simulink model "Revised_model"  (Simulink 10.3)
settings: Solver=ode3  StartTime=0.0  StopTime=12  FixedStep=ts  MaxStep=1e-4  RelTol=1e-3
undefined symbols (not defined in the file or in its folder): Ion, Lithium, sigbuilder_block, ts
libraries: spsMeanLib x9, spsSeriesRLCBranchLib x6, spsIGBTDiodeLib x4, pid_lib x4, spsPWMGeneratorDCDCLib x4, spsBatteryLib x2, spsCurrentMeasurementLib x2, spsControlledCurrentSourceLib x2, spsVoltageMeasurementLib x2, spsFirstOrderFilterLib x1, spsDiodeLib x1, spsIGBTLib x1
(part 1 of 2)
settings Model: Creator=Rodayna  LastModifiedBy=Aditya  SimulationMode=accelerator
settings DataIOCC: SaveFormat=Dataset  SignalLoggingSaveFormat=Dataset
settings OptimizationCC: ExpressionDepthLimit=128  LifeSpan=auto
settings DebuggingCC: UnderspecifiedInitializationDetection=Simplified  MergeDetectMultiDrivingBlocksExec=error  FcnCallInpInsideContextMsg=error  StateNameClashWarn=none  SFUnexpectedBacktrackingDiag=error  SFNoUnconditionalDefaultTransitionDiag=error  SFExecutionAtInitializationDiag=warning
settings HardwareCC: ProdBitPerPointer=64  ProdBitPerSizeT=64  ProdBitPerPtrDiffT=64  ProdLargestAtomicFloat=Float  ProdIntDivRoundTo=Zero  ProdEndianess=LittleEndian  ProdWordSize=64  ProdHWDeviceType=Intel->x86-64 (Windows64)
settings ModelReferenceCC: PropagateSignalLabelsOutOfModel=on
settings GRTTargetCC: TargetLangStandard=C99 (ISO)  CombineOutputUpdateFcns=on  GRTInterface=off
settings ConfigComp: CovMetricSettings=dwe  CovSaveCumulativeToWorkspaceVar=off  CovSaveSingleToWorkspaceVar=off  CovExternalEMLEnable=on
settings SimscapeCC: SimscapeNormalizeSystem=off

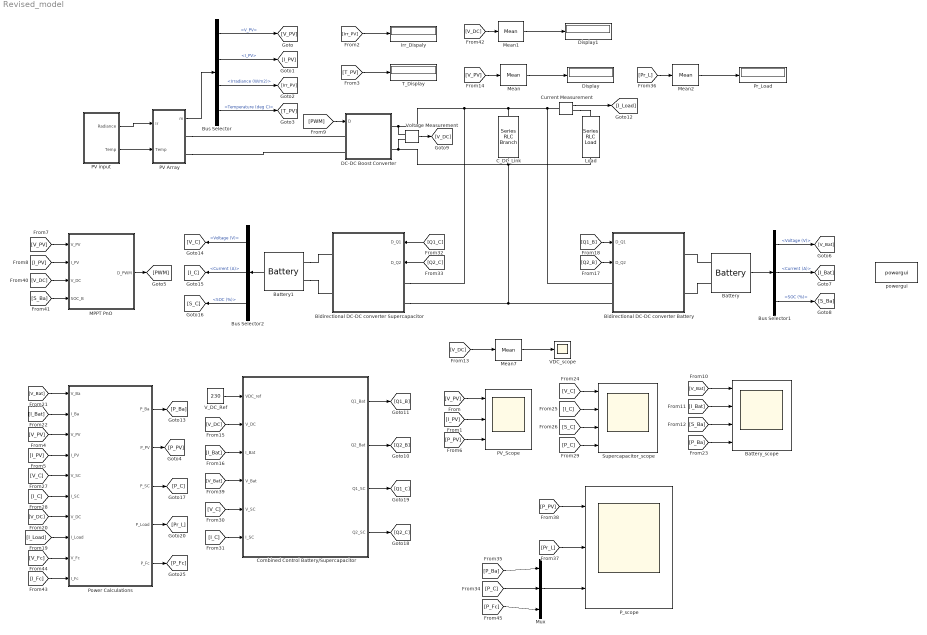
== system Revised_model ==
  Battery : spsBatteryLib/Battery  BatType=Lithium-Ion  ShowTempParam=off  ThermalPreset=no  ShowAgeParam=off  NomV=110  NomQ=150  SOC=50  Batt_Tr=0.1  PresetModel=on  MaxQ=150  MinV=82.5  FullV=128.0386  Dis_rate=65.2174  R=0.0073333  Normal_OP=135.6522  expZone="[118.8424      7.369565]"  current=[6.5 13 32.5]  Units=Time  Tci=20  NomT=20  T2=-30  MaxQ2=4.8  FullV2=7.1  Normal_OP2=5.655  expZone2="[6.58           1]"  Rca=0.6  ti=2000  Dp=0  Neq0=0  Tsim=1e6  Ta1=25  Qeol=5.4*0.9  Reol=0.013333*1.2  Char_age=[2.3478, 3]  Dis_age=[2.3478, 10]  N1=1500  N2=10500  N3=1000  N4=1400  Ta2=45  N5=950
  Battery1 : spsBatteryLib/Battery  BatType=Lithium-Ion  ShowTempParam=off  ThermalPreset=no  ShowAgeParam=off  NomV=154  NomQ=150  SOC=99  Batt_Tr=0.1  PresetModel=on  MaxQ=150  MinV=115.5  FullV=179.254  Dis_rate=65.2174  R=0.010267  Normal_OP=135.6522  expZone="[166.3794      7.369565]"  current=[6.5 13 32.5]  Units=Time  Tci=20  NomT=20  T2=-30  MaxQ2=4.8  FullV2=7.1  Normal_OP2=5.655  expZone2="[6.58           1]"  Rca=0.6  ti=2000  Dp=0  Neq0=0  Tsim=1e6  Ta1=25  Qeol=5.4*0.9  Reol=0.013333*1.2  Char_age=[2.3478, 3]  Dis_age=[2.3478, 10]  N1=1500  N2=10500  N3=1000  N4=1400  Ta2=45  N5=950
  "Battery_scope " : Scope  NumInputPorts=4
  Bidirectional DC-DC converter Battery : Subsystem
  Bidirectional DC-DC converter Supercapacitor : Subsystem
  Bus Selector : BusSelector  OutputSignals=V_PV,I_PV,Irradiance (W/m2),Temperature (deg C)
  Bus Selector1 : BusSelector  OutputSignals=Voltage (V),Current (A),SOC (%)
  Bus Selector2 : BusSelector  OutputSignals=Voltage (V),Current (A),SOC (%)
  C_DC_Link : spsSeriesRLCBranchLib/Series RLC Branch  LConnTagsString=__new0  RConnTagsString=__new0  BranchType=C  Resistance=1  Inductance=1e-3  SetiL0=off  InitialCurrent=0  Capacitance=3000e-6  Setx0=on  InitialVoltage=230  Measurements=None
  Combined Control Battery/Supercapacitor : Subsystem
  Current Measurement : spsCurrentMeasurementLib/Current Measurement  PhasorSimulation=off  OutputType=Complex  PSBequivalent=0
  DC-DC Boost Converter : Subsystem
  Display : Display
  Display1 : Display
  Irr_Dispaly : Display
  Load : spsSeriesRLCLoadLib/Series RLC Load  LConnTagsString=a  RConnTagsString=__new0  NominalVoltage=230  NominalFrequency=0.00001  ActivePower=10e3  InductivePower=0  CapacitivePower=0  Setx0=off  InitialVoltage=0  SetiL0=off  InitialCurrent=0  Measurements=None  LoadType=constant Z
  MPPT PnO : Subsystem
  Mean{,1..2,7} (4 alike) : spsMeanLib/Mean  Freq=60  Vinit=0  Ts=0
  Mux : Mux  Inputs=3
  PV Array : Subsystem  mask(PV array){ModuleType=BP Solar SX3190, Ncell=50, Nser=5, Npar=12, Voc=30.6021, Isc=8.5103, Vm=24.3003, Im=7.8294, TempC_Voc=-0.111, TempC_Isc=0.005532, TempC_Vmp=-0.114, TempC_Imp=-0.001566, Qd=1.25, Temperature=[0   25   50   75  100], Iph_Temp=[8.3797      8.5214       8.667      8.8096      8.9362], Isat_Temp=[1.1494e-09  4.3763e-08   9.524e-07  1.3432e-05  0.00013518], Rp_Temp=[479.1668      189.6748      120.6956      107.8176      267.7255], Rs_Temp=[0.24905     0.24841     0.25704     0.27792     0.31611], PlotVI_module=off, PlotVI_array=off, PlotVI_array_Temp=off, Ts=ts}
      mask prompts: ModuleType "Module type:"; Ncell "Number of cells per module:"; Nser "Number of series-connected  modules per string (Nser):"; Npar "Number of parallel strings (Npar):"; Voc "Open circuit voltage  Voc (V):"; Isc "Short-circuit current Isc (A):"; Vm "Voltage at maximum power point Vmp (V):"; Im "Current at maximum power point Imp (A):"; TempC_Voc "Temperature coefficient of Voc (V/deg.C)"; TempC_Isc "Temperature coefficient of Isc (A/deg.C)"; TempC_Vmp "Temperature coefficient of Vmp (V/deg.C)"; TempC_Imp "Temperature coefficient of Imp (A/deg.C"; Qd "Diode Quality factor"; Temperature "Cell temperature (degrees C)"; Iph_Temp "Photo-current source Iph  (A):"; Isat_Temp "Diode saturation current Isat (A):"; Rp_Temp "Parallel resistance Rp (ohms):"; Rs_Temp "Series resistance Rs (ohms):"; PlotVI_module "Display  I-V and  P-V characteristics of one module at 25 deg.C"; PlotVI_array "Display  I-V and  P-V characteristics of array at 25 deg.C"; PlotVI_array_Temp "Display  I-V and  P-V char. of array at 100W/m^2  for specified temperatures"; Ts "Sample time"
      mask help:
      | Model a PV array.
      |
      | PV array consists of Npar strings of modules connected in parallel, each string consisting of Nser modules connected in series.
      |
      | Input 1 = Sun irradiance (W/m^2)
      | Input 2 = Cell temperature (deg.C))
      |
      | Module specifications provided by manufacturer (Voc, Isc, Vmp, Imp) as well as temperature coefficients are listed under 'Module' Tab.
      | The four PV model parameters for one module (photo-generated current Iph, diode saturation current Isat, parallel resistance Rp and  series resistance Rs) are listed under the 'Model' Tab. These parameters are adusted to fit Voc, Isc, Vmp, Imp at specied cell temperatures listed under 'Module' Tab and assuming a given "diode quality factor" (Qd) for the semiconductor.
      |
      | Select a 'Module type' and then press Apply to see module parameters.
      | Note: Module characteristics are extracted from NREL System Advisor Model.
      mask init:
      | BlockName=gcb;
      | 
      | % Solar Modules Specifications
      | %=============================
      | %
      | Type=1;
      | SolarModuleSpec(Type).Desc= 'Kyocera KD135GX-LP';
      | SolarModuleSpec(Type).nCells= 36;
      | SolarModuleSpec(Type).Voc= 22.0999;
      | SolarModuleSpec(Type).Isc= 8.36955;
      | SolarModuleSpec(Type).Vmp= 17.7;
      | SolarModuleSpec(Type).Imp= 7.62959;
      | SolarModuleSpec(Type).TempC_Voc= -0.08;
      | SolarModuleSpec(Type).TempC_Isc= 0.005022;
      | SolarModuleSpec(Type).TempC_Vmp= -0.082;
      | SolarModuleSpec(Type).TempC_Imp= -0.001068;
      | SolarModuleSpec(Type).TempC= [0   25   50   75  100];
      | SolarModuleSpec(Type).Qd= 1.25;
      | SolarModuleSpec(Type).Iph= [8.2548      8.3863      8.5179      8.6475      8.7657];
      | SolarModuleSpec(Type).Isat= [1.0452e-09  4.0088e-08  8.7854e-07   1.246e-05  0.00012585];
      | SolarModuleSpec(Type).Rp= [124.2147      80.21788      61.82143      57.59975       93.2949];
      | SolarModuleSpec(Type).Rs= [0.16273     0.16086     0.16567     0.17914     0.20462];
      | SolarModuleSpec(Type).VT= [1.0586      1.1555      1.2525      1.3494      1.4463];
      | 
      | Type=2;
      | SolarModuleSpec(Type).Desc= 'Kyocera KD205GX-LP';
      | SolarModuleSpec(Type).nCells= 54;
      | SolarModuleSpec(Type).Voc= 33.1999;
      | SolarModuleSpec(Type).Isc= 8.35955;
      | SolarModuleSpec(Type).Vmp= 26.6;
      | SolarModuleSpec(Type).Imp= 7.70959;
      | SolarModuleSpec(Type).TempC_Voc= -0.12;
      | SolarModuleSpec(Type).TempC_Isc= 0.005016;
      | SolarModuleSpec(Type).TempC_Vmp= -0.123;
      | SolarModuleSpec(Type).TempC_Imp= -0.001079;
      | SolarModuleSpec(Type).TempC= [0   25   50   75  100];
      | SolarModuleSpec(Type).Qd= 1.5;
      | SolarModuleSpec(Type).Iph= [8.2611      8.3642      8.4897      8.6397      8.8494];
      | SolarModuleSpec(Type).Isat= [4.6184e-08  9.7399e-07  1.2856e-05  0.00011784  0.00080899];
      | SolarModuleSpec(Type).Rp= [1053.4598       1010.571      746.03259      733.82072      575.51725];
      | SolarModuleSpec(Type).Rs= [0.16179     0.15945     0.16818     0.19126     0.23373];
      | SolarModuleSpec(Type).VT= [1.9055      2.0799      2.2544      2.4289      2.6034];
      | 
      | Type=3;
      | SolarModuleSpec(Type).Desc= 'Mitsubishi PV-UD190MF5';
      | SolarModuleSpec(Type).nCells= 50;
      | SolarModuleSpec(Type).Voc= 30.8006;
      | SolarModuleSpec(Type).Isc= 8.23289;
      | SolarModuleSpec(Type).Vmp= 24.6999;
      | SolarModuleSpec(Type).Imp= 7.71272;
      | SolarModuleSpec(Type).TempC_Voc= -0.105;
      | SolarModuleSpec(Type).TempC_Isc= 0.004446;
      | SolarModuleSpec(Type).TempC_Vmp= -0.109;
      | SolarModuleSpec(Type).TempC_Imp= -0.0007713;
      | SolarModuleSpec(Type).TempC= [0   25   50   75  100];
      | SolarModuleSpec(Type).Qd= 1.25;
      | SolarModuleSpec(Type).Iph= [8.1758      8.2585      8.3644      8.4965      8.6704];
      | SolarModuleSpec(Type).Isat= [1.0882e-09  3.8061e-08  7.7001e-07  1.0166e-05  9.5622e-05];
      | SolarModuleSpec(Type).Rp= [760.17338      1011.1501      920.18116      953.25748       1044.703];
      | SolarModuleSpec(Type).Rs= [0.22154      0.2231     0.23302     0.25351     0.28829];
      | SolarModuleSpec(Type).VT= [1.4703      1.6049      1.7395      1.8742      2.0088];
      | 
      | Type=4;
      | SolarModuleSpec(Type).Desc= 'Sanyo HIP-225HDE1';
      | SolarModuleSpec(Type).nCells= 60;
      | SolarModuleSpec(Type).Voc= 41.7984;
      | SolarModuleSpec(Type).Isc= 7.13383;
      | SolarModuleSpec(Type).Vmp= 33.9;
      | SolarModuleSpec(Type).Imp= 6.63419;
      | SolarModuleSpec(Type).TempC_Voc= -0.105;
      | SolarModuleSpec(Type).TempC_Isc= 0.00214;
      | SolarModuleSpec(Type).TempC_Vmp= -0.101;
      | SolarModuleSpec(Type).TempC_Imp= -0.0006634;
      | SolarModuleSpec(Type).TempC= [0   25   50   75  100];
      | SolarModuleSpec(Type).Qd= 1.75;
      | SolarModuleSpec(Type).Iph= [7.1125      7.1668      7.2277      7.3002      7.3835];
      | SolarModuleSpec(Type).Isat= [1.0956e-07   1.322e-06  1.0873e-05  6.6227e-05  0.00031754];
      | SolarModuleSpec(Type).Rp= [1677.488      1798.4952      1967.0424      1956.9124      2053.1618];
      | SolarModuleSpec(Type).Rs= [0.19173     0.14196     0.10096    0.069476    0.049098];
      | SolarModuleSpec(Type).VT= [2.47      2.6962      2.9224      3.1486      3.3748];
      | 
      | Type=5;
      | SolarModuleSpec(Type).Desc= 'SunPower SPR-305-WHT';
      | SolarModuleSpec(Type).nCells= 96;
      | SolarModuleSpec(Type).Voc= 64.2;
      | SolarModuleSpec(Type).Isc= 5.96;
      | SolarModuleSpec(Type).Vmp= 54.7;
      | SolarModuleSpec(Type).Imp= 5.58;
      | SolarModuleSpec(Type).TempC_Voc= -0.177;
      | SolarModuleSpec(Type).TempC_Isc= 0.003516;
      | SolarModuleSpec(Type).TempC_Vmp= -0.186;
      | SolarModuleSpec(Type).TempC_Imp= -0.00212;
      | SolarModuleSpec(Type).TempC= [0   25   50   75  100];
      | SolarModuleSpec(Type).Qd= 1.25;
      | SolarModuleSpec(Type).Iph= [5.9045      5.9606      6.0494      6.1386      6.2292];
      | SolarModuleSpec(Type).Isat= [1.6236e-10  5.2622e-09  9.8888e-08  1.2201e-06  1.0769e-05];
      | SolarModuleSpec(Type).Rp= [1723.2701      819.13001       313.3225      186.86379      130.70398];
      | SolarModuleSpec(Type).Rs= [0.10187    0.083029    0.075997    0.085738      0.1163];
      | SolarModuleSpec(Type).VT= [2.8229      3.0814      3.3399      3.5984      3.8569];
      | 
      | Type=6;
      | SolarModuleSpec(Type).Desc= 'Suntech STP270S-24_Vb';
      | SolarModuleSpec(Type).nCells= 72;
      | SolarModuleSpec(Type).Voc= 44.4999;
      | SolarModuleSpec(Type).Isc= 8.19978;
      | SolarModuleSpec(Type).Vmp= 35;
      | SolarModuleSpec(Type).Imp= 7.70979;
      | SolarModuleSpec(Type).TempC_Voc= -0.1504;
      | SolarModuleSpec(Type).TempC_Isc= 0.004969;
      | SolarModuleSpec(Type).TempC_Vmp= -0.1567;
      | SolarModuleSpec(Type).TempC_Imp= 0.0001234;
      | SolarModuleSpec(Type).TempC= [0   25   50   75  100];
      | SolarModuleSpec(Type).Qd= 1.25;
      | SolarModuleSpec(Type).Iph= [8.1345      8.2466      8.3792      8.5437      8.7583];
      | SolarModuleSpec(Type).Isat= [1.0212e-09   3.569e-08  7.2273e-07  9.5489e-06  8.9954e-05];
      | SolarModuleSpec(Type).Rp= [1505.3115      1827.4593      2300.9307      2164.0121      1763.1975];
      | SolarModuleSpec(Type).Rs= [0.4218     0.42722     0.44553     0.48023      0.5376];
      | SolarModuleSpec(Type).VT= [2.1172      2.3111      2.5049      2.6988      2.8927];
      | 
      | Type=7;
      | SolarModuleSpec(Type).Desc= 'Canadian Solar CS5P-220M';
      | SolarModuleSpec(Type).nCells= 96;
      | SolarModuleSpec(Type).Voc= 59.2618;
      | SolarModuleSpec(Type).Isc= 5.09261;
      | SolarModuleSpec(Type).Vmp= 48.3159;
      | SolarModuleSpec(Type).Imp= 4.54758;
      | SolarModuleSpec(Type).TempC_Voc= -0.217;
      | SolarModuleSpec(Type).TempC_Isc= 0.002022;
      | SolarModuleSpec(Type).TempC_Vmp= -0.2355;
      | SolarModuleSpec(Type).TempC_Imp= 0.0008231;
      | SolarModuleSpec(Type).TempC= [0   25   50   75  100];
      | SolarModuleSpec(Type).Qd= 1.5;
      | SolarModuleSpec(Type).Iph= [5.046       5.098      5.1493      5.1959      5.3427];
      | SolarModuleSpec(Type).Isat= [2.4207e-08  5.3103e-07  7.2907e-06  6.9747e-05  0.00049283];
      | SolarModuleSpec(Type).Rp= [222.52442      235.76261      303.25525      1307.0023      2378.4408];
      | SolarModuleSpec(Type).Rs= [0.17441     0.24807     0.36157     0.52616      0.7509];
      | SolarModuleSpec(Type).VT= [3.3875      3.6977      4.0079      4.3181      4.6283];
      | 
      | Type=8;
      | SolarModuleSpec(Type).Desc= 'BP Solar SX3190';
      | SolarModuleSpec(Type).nCells= 50;
      | SolarModuleSpec(Type).Voc= 30.6021;
      | SolarModuleSpec(Type).Isc= 8.51029;
      | SolarModuleSpec(Type).Vmp= 24.3003;
      | SolarModuleSpec(Type).Imp= 7.82945;
      | SolarModuleSpec(Type).TempC_Voc= -0.111;
      | SolarModuleSpec(Type).TempC_Isc= 0.005532;
      | SolarModuleSpec(Type).TempC_Vmp= -0.114;
      | SolarModuleSpec(Type).TempC_Imp= -0.001566;
      | SolarModuleSpec(Type).TempC= [0   25   50   75  100];
      | SolarModuleSpec(Type).Qd= 1.25;
      | SolarModuleSpec(Type).Iph= [8.3797      8.5214       8.667      8.8096      8.9362];
      | SolarModuleSpec(Type).Isat= [1.1494e-09  4.3763e-08   9.524e-07  1.3432e-05  0.00013518];
      | SolarModuleSpec(Type).Rp= [479.1668      189.6748      120.6956      107.8176      267.7255];
      | SolarModuleSpec(Type).Rs= [0.24905     0.24841     0.25704     0.27792     0.31611];
      | SolarModuleSpec(Type).VT= [1.4703      1.6049      1.7395      1.8742      2.0088];
      | 
      | Type=9;
      | SolarModuleSpec(Type).Desc= 'First Solar FS-272';
      | SolarModuleSpec(Type).nCells= 116;
      | SolarModuleSpec(Type).Voc= 94.5738;
      | SolarModuleSpec(Type).Isc= 1.18103;
      | SolarModuleSpec(Type).Vmp= 70.558;
      | SolarModuleSpec(Type).Imp= 1.01088;
      | SolarModuleSpec(Type).TempC_Voc= -0.269;
      | SolarModuleSpec(Type).TempC_Isc= 0.0005433;
      | SolarModuleSpec(Type).TempC_Vmp= -0.206;
      | SolarModuleSpec(Type).TempC_Imp= -0.0003538;
      | SolarModuleSpec(Type).TempC= [0   25   50   75  100];
      | SolarModuleSpec(Type).Qd= 3;
      | SolarModuleSpec(Type).Iph= [1.1706      1.1841      1.1969       1.209      1.2204];
      | SolarModuleSpec(Type).Isat= [4.7807e-06   2.871e-05  0.00013082  0.00048055    0.001489];
      | SolarModuleSpec(Type).Rp= [2555.993      1859.5401      1459.3976      1213.5712      1072.4965];
      | SolarModuleSpec(Type).Rs= [6.9861      4.7977      2.7078     0.74048           0];
      | SolarModuleSpec(Type).VT= [8.1864      8.93607      9.68574      10.4354      11.1851];
      | 
      | Type=10;
      | SolarModuleSpec(Type).Desc= 'SunPower 128-cell Module';
      | SolarModuleSpec(Type).nCells= 128;
      | SolarModuleSpec(Type).Voc= 85.2983;
      | SolarModuleSpec(Type).Isc= 5.8675;
      | SolarModuleSpec(Type).Vmp= 72.8992;
      | SolarModuleSpec(Type).Imp= 5.48769;
      | SolarModuleSpec(Type).TempC_Voc= -0.2664;
      | SolarModuleSpec(Type).TempC_Isc= 0.001837;
      | SolarModuleSpec(Type).TempC_Vmp= -0.276;
      | SolarModuleSpec(Type).TempC_Imp= -0.00169;
      | SolarModuleSpec(Type).TempC= [0   25   50   75  100];
      | SolarModuleSpec(Type).Qd= 1.5;
      | SolarModuleSpec(Type).Iph= [5.8403      5.8693      5.9126      5.9583      6.0069];
      | SolarModuleSpec(Type).Isat= [8.3639e-09  1.7905e-07  2.3847e-06  2.1965e-05  0.00015113];
      | SolarModuleSpec(Type).Rp= [3739.8323      3390.2471      1695.8516      1327.4043      1910.4252];
      | SolarModuleSpec(Type).Rs= [0  0  0  0  0];
      | SolarModuleSpec(Type).VT= [4.5166      4.9302      5.3439      5.7575      6.1711];
      | 
      | 
      | %-------------------------------------------------------------------------
      | 
      | Type=strmatch(ModuleType,char(SolarModuleSpec.Desc));
      | 
      | % Write module prameters inside mask
      | %===================================
      | set_param(BlockName,'Ncell',num2str(SolarModuleSpec(Type).nCells));
      | set_param(BlockName,'Voc',num2str(SolarModuleSpec(Type).Voc));
      | set_param(BlockName,'Isc',num2str(SolarModuleSpec(Type).Isc));
      | set_param(BlockName,'Vm',num2str(SolarModuleSpec(Type).Vmp));
      | set_param(BlockName,'Im',num2str(SolarModuleSpec(Type).Imp));
      | set_param(BlockName,'TempC_Voc',num2str(SolarModuleSpec(Type).TempC_Voc));
      | set_param(BlockName,'TempC_Isc',num2str(SolarModuleSpec(Type).TempC_Isc));
      | set_param(BlockName,'TempC_Vmp',num2str(SolarModuleSpec(Type).TempC_Vmp));
      | set_param(BlockName,'TempC_Imp',num2str(SolarModuleSpec(Type).TempC_Imp));
      | 
      | set_param(BlockName,'Qd',num2str(SolarModuleSpec(Type).Qd));
      | 
      | set_param(BlockName,'Temperature',['[',num2str(SolarModuleSpec(Type).TempC),']']);
      | set_param(BlockName,'Iph_Temp',['[',num2str(SolarModuleSpec(Type).Iph),']']);
      | set_param(BlockName,'Isat_Temp',['[',num2str(SolarModuleSpec(Type).Isat),']']);
      | set_param(BlockName,'Rp_Temp',['[',num2str(SolarModuleSpec(Type).Rp),']']);
      | set_param(BlockName,'Rs_Temp',['[',num2str(SolarModuleSpec(Type).Rs),']']);
      | 
      | TC=25; % standard test temperature (deg. C)
      | T=273+TC; %(Kelvin)
      | nT=find(SolarModuleSpec(Type).TempC==TC);
      | 
      | % Array model parameters
      | %=======================
      | % Qd=SolarModuleSpec(Type).Qd;
      | % k= 1.3806e-23; % Boltzman constant (J.K^-1)
      | % q=1.6022e-19;  % electron charge  (C)
      | % VT=k*T/q*nCells*Qd;
      | VT=SolarModuleSpec(Type).VT(nT);Iph=SolarModuleSpec(Type).Iph(nT); 
      | 
      | TempC=SolarModuleSpec(Type).TempC;
      | Iph_array=SolarModuleSpec(Type).Iph*Npar;
      | Isat_array=SolarModuleSpec(Type).Isat*Npar;
      | VT_array=SolarModuleSpec(Type).VT*Nser;
      | Rs_array=SolarModuleSpec(Type).Rs*Nser/Npar;
      | Rp_array=SolarModuleSpec(Type).Rp*Nser/Npar;
      | 
      | % Used to determine initial value of Boost Control (MPPT)
      | % assignin('base','Vm_Init',Vm*Nser);
      | %
      | % Plot module and array I-V & P-V characteristics for different irradiances
      | % =========================================================================
      | if PlotVI_module || PlotVI_array 
      |     Voc=SolarModuleSpec(Type).Voc; 
      |     Isc=SolarModuleSpec(Type).Isc; 
      |     Vm=SolarModuleSpec(Type).Vmp;  
      |     Im=SolarModuleSpec(Type).Imp;
      |     
      |     load_system('PV_model_Param');
      |     
      |     assignin('base','Voc',Voc);
      |     assignin('base','Isc',Isc);
      |     assignin('base','Rs',SolarModuleSpec(Type).Rs(nT));
      |     assignin('base','Rp',SolarModuleSpec(Type).Rp(nT));
      |     assignin('base','Isat',SolarModuleSpec(Type).Isat(nT));
      |     assignin('base','VT',SolarModuleSpec(Type).VT(nT));
      |    
      |     if PlotVI_module,
      |         F1=figure('Name','I-V and P-V characteristics of one module at 25 deg.C');  
      |     end
      |     if PlotVI_array
      |         F2=figure('Name','I-V and P-V characteristics of array at 25 deg.C'); 
      |     end
      | 
      |     for ksun=1:-0.25:0.25
      |         assignin('base','Iph',SolarModuleSpec(Type).Iph(nT)*ksun);
      |         sim('PV_model_Param');
      |         n=find(I_PV>=0);
      |         I_PV=I_PV(n);
      |         V_PV=V_PV(n);
      |         P_PV=V_PV.*I_PV;
      |         
      |         % Plot I-V & P-V characteristics of one module
      |         %=============================================
      |         if PlotVI_module
      |             figure(F1);
      |             subplot(211)
      |             if ksun==1
      |                 plot(V_PV,I_PV,'b',[0  Vm Voc], [Isc Im 0],'ro')
      |                 text(Voc/15,Isc*1.1,'1 kW/m^2')
      |                 hold on
      |                 grid
      |             else
      |                 plot(V_PV,I_PV,'--m')
      |                 text(Voc/15, Isc*(ksun+0.1) , sprintf('%g kW/m^2',ksun))
      |             end
      | 
      |             subplot(212) 
      |             if ksun==1
      |                 plot(V_PV,P_PV,'b',[0  Vm Voc], [0 Im*Vm 0],'ro')
      |                 text(Vm*1.02,Vm*Im,'1 kW/m^2')
      |                 hold on
      |                 grid
      |             else
      |                 n= find(P_PV==max(P_PV));
      |                 plot(V_PV,P_PV,'--m', V_PV(n) , P_PV(n),'mo')
      |                 text(Vm*1.02, Vm*Im*ksun, sprintf('%g kW/m^2',ksun))
      |             end
      |             subplot(211)
      |             ylabel('Current (A)')
      |             xlabel('Voltage (V)')
      |             title(sprintf('Module type: %s',SolarModuleSpec(Type).Desc))
      |             axis_xy=axis;
      |             axis_xy(4)=Isc*1.2;
      |             axis(axis_xy);
      |             
      |             subplot(212)
      |             ylabel('Power (W)')
      |             xlabel('Voltage (V)')
      |             axis_xy=axis;
      |             axis_xy(4)=Vm*Im*1.2;
      |             axis(axis_xy);
      |                   
      |             set_param(BlockName,'PlotVI_module', 'off')
      |         end
      |         
      |         % Plot I-V & P-V characteristics of array
      |         %========================================
      |         if PlotVI_array
      |             figure(F2);
      |             subplot(211)
      |             if ksun==1
      |                 plot(V_PV*Nser,I_PV*Npar,'b',[0  Vm Voc]*Nser, [Isc Im 0]*Npar,'ro')
      |                 text(Voc/15*Nser,Isc*1.1*Npar,'1 kW/m^2')
      |                 hold on
      |                 grid
      |             else
      |                 plot(V_PV*Nser,I_PV*Npar,'--m')
      |                 text(Voc*Nser/15, Isc*Npar*(ksun+0.1) , sprintf('%g kW/m^2',ksun))
      |             end
      |            
      |             subplot(212)
      |             if ksun==1
      |                 plot(V_PV*Nser,P_PV*Nser*Npar,'b',[0  Vm Voc]*Nser, [0 Im*Vm 0]*Nser*Npar,'ro')
      |                 text(Vm*Nser*1.02,Vm*Im*Nser*Npar,'1 kW/m^2')
      |                 hold on
      |                 grid
      |             else
      |                 n= find(P_PV==max(P_PV));
      |                 plot(V_PV*Nser,P_PV*Nser*Npar,'--m', V_PV(n)*Nser , P_PV(n)*Nser*Npar,'mo')
      |                 text(Vm*Nser*1.02, Vm*Im*Nser*Npar*ksun, sprintf('%g kW/m^2',ksun))
      |             end 
      |             subplot(211)
      |             ylabel('Current (A)')
      |             xlabel('Voltage (V)')
      |             title(sprintf('Array type: %s; %d series modules; %d parallel strings',SolarModuleSpec(Type).Desc,Nser,Npar));
      |             axis_xy=axis;
      |             axis_xy(4)=Isc*Npar*1.2;
      |             axis(axis_xy);
      |             
      |             subplot(212)
      |             ylabel('Power (W)')
      |             xlabel('Voltage (V)')
      |             xis_xy=axis;
      |             axis_xy(4)=Vm*Im*Nser*Npar*1.2;
      |             axis(axis_xy);
      |             
      |             set_param(BlockName,'PlotVI_array', 'off')
      |         end
      |         
      |     end  
      | end
      | 
      | %%  Plot array V-I & P_V characteristics for different temperatures
      | % =================================================================
      | if PlotVI_array_Temp
      |     F3=figure('Name',' I-V and P-V characteristics of array at 1000 W/m^2');
      |     load_system('PV_model_Param');
      |     for ktemp=1:length(TempC)
      |         DeltaT=TempC(ktemp)-25;
      |         Voc=SolarModuleSpec(Type).Voc + SolarModuleSpec(Type).TempC_Voc*DeltaT;
      |         Isc=SolarModuleSpec(Type).Isc + SolarModuleSpec(Type).TempC_Isc*DeltaT;
      |         Vm=SolarModuleSpec(Type).Vmp  + SolarModuleSpec(Type).TempC_Vmp*DeltaT;
      |         Im=SolarModuleSpec(Type).Imp  + SolarModuleSpec(Type).TempC_Imp*DeltaT;
      | 
      |         assignin('base','Voc',Voc)
      |         assignin('base','Isc',Isc)
      |         assignin('base','Iph',SolarModuleSpec(Type).Iph(ktemp));
      |         assignin('base','Isat',SolarModuleSpec(Type).Isat(ktemp));
      |         assignin('base','Rs',SolarModuleSpec(Type).Rs(ktemp));
      |         assignin('base','Rp',SolarModuleSpec(Type).Rp(ktemp));
      |         assignin('base','VT',SolarModuleSpec(Type).VT(ktemp));
      |         
      |         sim('PV_model_Param');
      |         n=find(I_PV>=0);
      |         I_PV=I_PV(n);
      |         V_PV=V_PV(n);
      |         P_PV=V_PV.*I_PV;
      | 
      |         subplot(211)
      |         if TempC(ktemp)==25
      |             plot(V_PV*Nser,I_PV*Npar,'b',[0  Vm Voc]*Nser, [Isc Im 0]*Npar,'ro')
      |             text(Voc*Nser*0.95, Isc*Npar/10*(1+ktemp) , sprintf('%g ^oC',TempC(ktemp)))
      |             %hold on
      |             grid
      |         else
      |             plot(V_PV*Nser,I_PV*Npar,'--m',[0  Vm Voc]*Nser, [Isc Im 0]*Npar,'mo')
      |             text(Voc*Nser*0.95, Isc*Npar/10*(1+ktemp) , sprintf('%g ^oC',TempC(ktemp)))
      |         end
      |         if ktemp==1, hold on; end
      | 
      |         subplot(212) 
      |         if TempC(ktemp)==25
      |             plot(V_PV*Nser,P_PV*Nser*Npar,'b',[0  Vm Voc]*Nser, [0 Im*Vm 0]*Nser*Npar,'ro')
      |             text(Vm*Nser, 0.9*Vm*Im*Nser*Npar , sprintf('%g ^oC',TempC(ktemp)))
      |             %hold on
      |             grid
      |         else
      |             n= find(P_PV==max(P_PV));
      |             plot(V_PV*Nser,P_PV*Nser*Npar,'--m', V_PV(n)*Nser , P_PV(n)*Nser*Npar,'mo')
      |             text(Vm*Nser, 0.9*Vm*Im*Nser*Npar , sprintf('%g ^oC',TempC(ktemp)))
      |         end
      |         if ktemp==1, hold on; end
      |     end
      |         
      |     subplot(211)
      |     ylabel('Current (A)')
      |     xlabel('Voltage (V)')
      |     title(sprintf('Array type: %s; %d series modules; %d parallel strings',SolarModuleSpec(Type).Desc,Nser,Npar));
      |     subplot(212)
      |     ylabel('Power (W)')
      |     xlabel('Voltage (V)')
      |     set_param(BlockName,'PlotVI_array_Temp', 'off')
      | end
      mask TypeOptions ModuleType: BP Solar SX3190 | Canadian Solar CS5P-220M | First Solar FS-272 | Kyocera KD135GX-LP | Kyocera KD205GX-LP | Mitsubishi PV-UD190MF5 | Sanyo HIP-225HDE1 | SunPower SPR-305-WHT | SunPower SPR-400-WHT | Suntech STP270S-24_Vb
      mask Display: image(imread('panel.jpg'))
  PV input : Subsystem  Tag=STV Subsys  LoadFcn=sigbuilder_block('load');  StartFcn=sigbuilder_block('start');  StopFcn=sigbuilder_block('stop');  ClipboardFcn=sigbuilder_block('clipboard');  mask(Sigbuilder block){tuvar=[0:10]}
      mask help: Simulink:masks:SigbuilderBlock_MD
      mask init:
      | if ~strcmp(get_param(bdroot(gcbh),'SimulationStatus'),'stopped') tuvar = sigbuilder_block('maskInit'); end
      settings: CopyFcn=sigbuilder_block('copy');  DeleteFcn=sigbuilder_block('delete');  ModelCloseFcn=sigbuilder_block('modelClose');  PreSaveFcn=sigbuilder_block('preSave');  PauseFcn=sigbuilder_block('pause');  ContinueFcn=sigbuilder_block('continue');  NameChangeFcn=sigbuilder_block('namechange');  OpenFcn=sigbuilder_block('open',[437.25 117.75 550.5 394.5 ]);  CloseFcn=sigbuilder_block('close');
      mask Display: plot(0, 0, 100, 100,[2, 2, 32, 32, 2], [68, 8, 8, 68, 68],[32, 2], [38, 38], [32, 19, 2],[53, 60, 44], [32, 17, 17, 2],[16, 16, 31, 31]);txt = getActiveGroup(gcbh);text(2, 100, txt,'verticalAlignment', 'top');
  PV_Scope : Scope  NumInputPorts=3
  P_scope : Scope  NumInputPorts=3
  Power Calculations : Subsystem
  Pr_Load : Display
  Supercapacitor_scope : Scope  NumInputPorts=4
  T_Display : Display
  VDC_scope : Scope
  V_DC_Ref : Constant  Value=230
  Voltage Measurement : spsVoltageMeasurementLib/Voltage Measurement  PhasorSimulation=off  OutputType=Complex  PSBequivalent=0
  powergui : spspowerguiLib/powergui  Priority=1  SimulationMode=Discrete  SampleTime=ts  frequency=60  Iterations=50  frequencyindice=0  Pbase=100e6  ErrMax=1e-4  UnitsV=kV  UnitsW=MW  buscounter=0  FunctionMessages=off  echomessages=off  EnableUseOfTLC=off  CurrentSourceSwitches=off  DisableSnubberDevices=off  DisableRonSwitches=off  DisableVfSwitches=off  DisplayEquations=off  AutomaticDiscreteSolvers=off  SolverType=Tustin/Backward Euler (TBE)  Interpol=off  ExternalGateDelay=off  methode=off  Ts=100  x0status=blocks  SPID=on  SwTol=0  HookPort=off  NonlinearTolerance=1e-4  nMaxIteration=100  ContinueOnMaxIteration=off  RestoreLinks=warning  ResistiveCurrentMeasurement=off  Frange=[0:2:500]  Ylog=off  Xlog=on  ShowGrid=off  save=off  variable=ZData  structure=0  ZoomFFT=off  StartTime=0.0  cycles=1  DisplayStyle=1  fundamental=60  FreqAxis=off  MaxFrequency=1000  frequencyindicesteady=1  RmsSteady=1  display=off
  wires:
  PV Array/1(m) -> Bus Selector/1
  Bus Selector/1 -> [V_PV]  "<V_PV>"
  Bus Selector/2 -> [I_PV]  "<I_PV>"
  Bus Selector/3 -> [Irr_PV]  "<Irradiance (W/m2)>"
  Bus Selector/4 -> [T_PV]  "<Temperature (deg C)>"
  [Irr_PV] -> Irr_Dispaly/1
  [T_PV] -> T_Display/1
  [PWM] -> DC-DC Boost Converter/1(D)
  [V_PV] -> MPPT PnO/1(V_PV)
  [I_PV] -> MPPT PnO/2(I_PV)
  MPPT PnO/1(D_PWM) -> [PWM]
  Battery/1 -> Bus Selector1/1
  Bus Selector1/1 -> [V_Bat]  "<Voltage (V)>"
  Bus Selector1/3 -> [S_Ba]  "<SOC (%)>"
  Bus Selector1/2 -> [I_Bat]  "<Current (A)>"
  Voltage Measurement/1 -> [V_DC]
  [Q2_B] -> Bidirectional DC-DC converter Battery/2(D_Q2)
  [Q1_B] -> Bidirectional DC-DC converter Battery/1(D_Q1)
  Current Measurement/1 -> [I_Load]
  Mean/1 -> Display/1
  [V_PV] -> Mean/1
  Mean1/1 -> Display1/1
  Battery1/1 -> Bus Selector2/1
  Bus Selector2/1 -> [V_C]  "<Voltage (V)>"
  Bus Selector2/2 -> [I_C]  "<Current (A)>"
  Bus Selector2/3 -> [S_C]  "<SOC (%)>"
  [Q1_C] -> Bidirectional DC-DC converter Supercapacitor/1(D_Q1)
  [Q2_C] -> Bidirectional DC-DC converter Supercapacitor/2(D_Q2)
  Mean2/1 -> Pr_Load/1
  [Pr_L] -> Mean2/1
  PV input/2(Temp) -> PV Array/2(Temp)
  V_DC_Ref/1 -> Combined Control Battery/Supercapacitor/1(VDC_ref)
  [V_DC] -> Combined Control Battery/Supercapacitor/2(V_DC)
  [I_Bat] -> Combined Control Battery/Supercapacitor/3(I_Bat)
  [V_Bat] -> Combined Control Battery/Supercapacitor/4(V_Bat)
  [V_C] -> Combined Control Battery/Supercapacitor/5("V_SC ")
  [I_C] -> Combined Control Battery/Supercapacitor/6(I_SC)
  Combined Control Battery/Supercapacitor/1(Q1_Bat) -> [Q1_B]
  Combined Control Battery/Supercapacitor/2(Q2_Bat) -> [Q2_B]
  Combined Control Battery/Supercapacitor/3(Q1_SC) -> [Q1_C]
  Combined Control Battery/Supercapacitor/4(Q2_SC) -> [Q2_C]
  PV input/1(Radiance) -> PV Array/1(Ir)
  [V_DC] -> MPPT PnO/3(V_DC)
  [S_Ba] -> MPPT PnO/4(SOC_B)
  [V_DC] -> Mean1/1
  [P_C] -> Supercapacitor_scope/4
  [S_C] -> Supercapacitor_scope/3
  [I_C] -> Supercapacitor_scope/2
  [V_C] -> Supercapacitor_scope/1
  [P_Ba] -> "Battery_scope "/4
  [S_Ba] -> "Battery_scope "/3
  [V_Bat] -> "Battery_scope "/1
  [I_Bat] -> "Battery_scope "/2
  [P_PV] -> PV_Scope/3
  [I_PV] -> PV_Scope/2
  [V_PV] -> PV_Scope/1
  Mean7/1 -> VDC_scope/1
  [V_DC] -> Mean7/1
  [I_PV] -> Power Calculations/4(I_PV)
  Power Calculations/3(P_SC) -> [P_C]
  Power Calculations/1(P_Ba) -> [P_Ba]
  Power Calculations/2(P_PV) -> [P_PV]
  [V_DC] -> Power Calculations/7(V_DC)
  [I_C] -> Power Calculations/6(I_SC)
  [V_C] -> Power Calculations/5(V_SC)
  [V_Bat] -> Power Calculations/1(V_Ba)
  Power Calculations/4(P_Load) -> [Pr_L]
  [I_Load] -> Power Calculations/8(I_Load)
  [V_PV] -> Power Calculations/3(V_PV)
  [I_Bat] -> Power Calculations/2(I_Ba)
  [P_PV] -> P_scope/1
  Mux/1 -> P_scope/3
  [P_C] -> Mux/2
  [Pr_L] -> P_scope/2
  [P_Ba] -> Mux/1
  [V_Fc] -> Power Calculations/9(V_Fc)
  [I_Fc] -> Power Calculations/10(I_Fc)
  Power Calculations/5(P_Fc) -> [P_Fc]
  [P_Fc] -> Mux/3
  connections:
  PV Array/RConn2 -- DC-DC Boost Converter/LConn2
  Voltage Measurement/LConn2 -- C_DC_Link/RConn1 -- Bidirectional DC-DC converter Supercapacitor/LConn2 -- Bidirectional DC-DC converter Battery/LConn2 -- Load/RConn1 -- DC-DC Boost Converter/RConn2
  Battery/LConn2 -- Bidirectional DC-DC converter Battery/RConn2
  PV Array/RConn1 -- DC-DC Boost Converter/LConn1
  Battery1/LConn1 -- Bidirectional DC-DC converter Supercapacitor/RConn1
  Battery1/LConn2 -- Bidirectional DC-DC converter Supercapacitor/RConn2
  Battery/LConn1 -- Bidirectional DC-DC converter Battery/RConn1
  Current Measurement/RConn1 -- Load/LConn1
  C_DC_Link/LConn1 -- Current Measurement/LConn1 -- Bidirectional DC-DC converter Battery/LConn1 -- Bidirectional DC-DC converter Supercapacitor/LConn1 -- Voltage Measurement/LConn1 -- DC-DC Boost Converter/RConn1

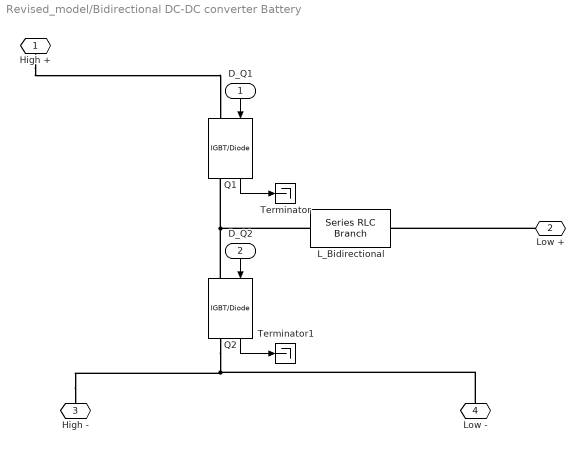
== system Revised_model/Bidirectional DC-DC converter Battery ==
  D_Q1 : Inport
  D_Q2 : Inport  Port=2
  L_Bidirectional : spsSeriesRLCBranchLib/Series RLC Branch  LConnTagsString=__new0  RConnTagsString=__new0  BranchType=RL  Resistance=0.05  Inductance=0.3e-3  SetiL0=off  InitialCurrent=0  Capacitance=1e-6  Setx0=off  InitialVoltage=0  Measurements=None
  Q1 : spsIGBTDiodeLib/IGBT//Diode  Ron=1e-3  Rs=1e5  Cs=inf  Measurements=on
  Q2 : spsIGBTDiodeLib/IGBT//Diode  Ron=1e-3  Rs=1e5  Cs=inf  Measurements=on
  Terminator : Terminator
  Terminator1 : Terminator
  High + : PMIOPort  Side=Left
  Low + : PMIOPort  Port=2  Side=Right
  High - : PMIOPort  Port=3  Side=Left
  Low - : PMIOPort  Port=4  Side=Right
  wires:
  D_Q2/1 -> Q2/1
  D_Q1/1 -> Q1/1
  Q1/1 -> Terminator/1
  Q2/1 -> Terminator1/1
  connections:
  High -/RConn1 -- Low -/RConn1 -- Q2/RConn1
  High +/RConn1 -- Q1/LConn1
  Low +/RConn1 -- L_Bidirectional/RConn1
  Q2/LConn1 -- L_Bidirectional/LConn1 -- Q1/RConn1

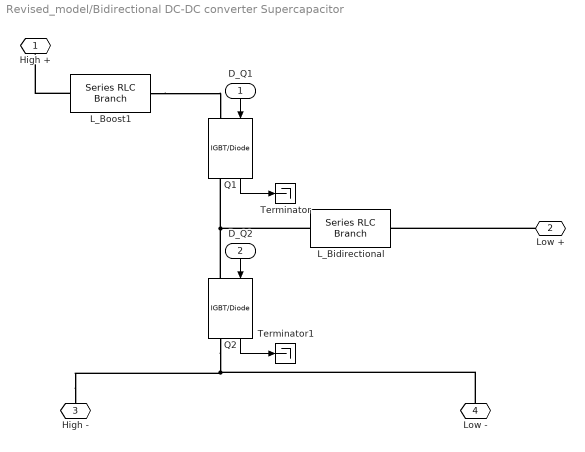
== system Revised_model/Bidirectional DC-DC converter Supercapacitor ==
  D_Q1 : Inport
  D_Q2 : Inport  Port=2
  L_Bidirectional : spsSeriesRLCBranchLib/Series RLC Branch  LConnTagsString=__new0  RConnTagsString=__new0  BranchType=RL  Resistance=0.05  Inductance=0.355e-3  SetiL0=off  InitialCurrent=0  Capacitance=1e-6  Setx0=off  InitialVoltage=0  Measurements=None
  L_Boost1 : spsSeriesRLCBranchLib/Series RLC Branch  LConnTagsString=__new0  RConnTagsString=__new0  BranchType=L  Resistance=0.05  Inductance=1.5e-3  SetiL0=off  InitialCurrent=0  Capacitance=1e-6  Setx0=off  InitialVoltage=0  Measurements=None
  Q1 : spsIGBTDiodeLib/IGBT//Diode  Ron=1e-3  Rs=1e5  Cs=inf  Measurements=on
  Q2 : spsIGBTDiodeLib/IGBT//Diode  Ron=1e-3  Rs=1e5  Cs=inf  Measurements=on
  Terminator : Terminator
  Terminator1 : Terminator
  High + : PMIOPort  Side=Left
  Low + : PMIOPort  Port=2  Side=Right
  High - : PMIOPort  Port=3  Side=Left
  Low - : PMIOPort  Port=4  Side=Right
  wires:
  D_Q2/1 -> Q2/1
  D_Q1/1 -> Q1/1
  Q1/1 -> Terminator/1
  Q2/1 -> Terminator1/1
  connections:
  High -/RConn1 -- Low -/RConn1 -- Q2/RConn1
  Low +/RConn1 -- L_Bidirectional/RConn1
  Q2/LConn1 -- L_Bidirectional/LConn1 -- Q1/RConn1
  L_Boost1/RConn1 -- Q1/LConn1
  L_Boost1/LConn1 -- High +/RConn1

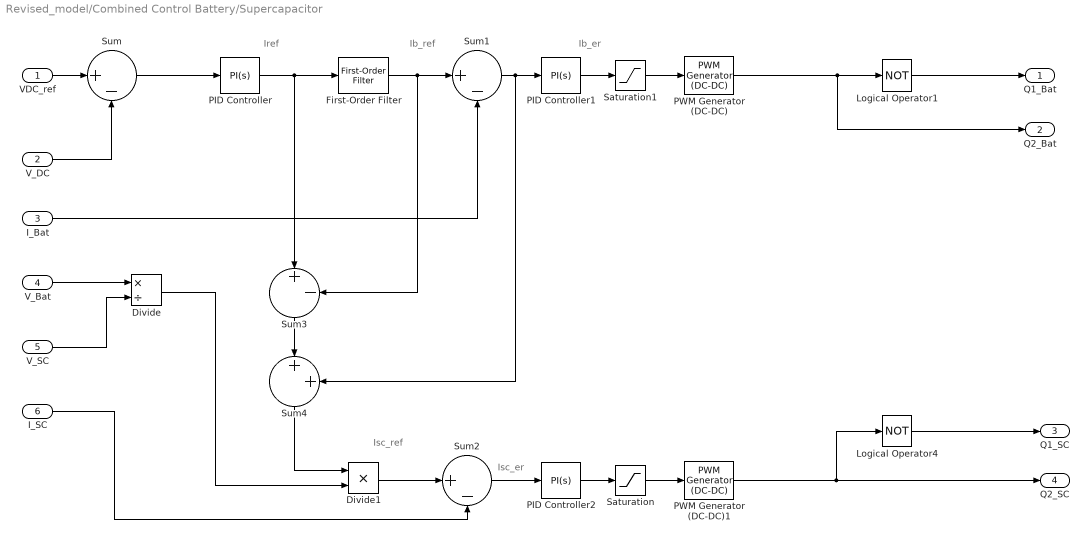
== system Revised_model/Combined Control Battery/Supercapacitor ==
  note: Isc_er
  note: Isc_ref
  note: Ib_er
  note: Ib_ref
  note: Iref
  VDC_ref : Inport
  V_DC : Inport  Port=2
  I_Bat : Inport  Port=3
  V_Bat : Inport  Port=4
  "V_SC " : Inport  Port=5
  I_SC : Inport  Port=6
  Divide : Product  Inputs=*/
  Divide1 : Product  Inputs=**
  First-Order Filter : spsFirstOrderFilterLib/First-Order Filter  FilterType=Lowpass  Tc=0.015  Ts=0  Initialize=off  Vac_Init=[0, 0, 60]  Vdc_Init=0  PlotResponse=off  FreqRange="[0,  200,  1]"
  Logical Operator1 : Logic  Operator=NOT  AllPortsSameDT=off  OutDataTypeStr=boolean
  Logical Operator4 : Logic  Operator=NOT  AllPortsSameDT=off  OutDataTypeStr=boolean
  PID Controller : pid_lib/PID Controller  Controller=PI  Form=Parallel  TimeDomain=Continuous-time  UseExternalTs=off  SampleTime=-1  IntegratorMethod=Forward Euler  FilterMethod=Forward Euler  ControllerParametersSource=internal  P=1.477  I=3077  D=0  UseFilter=on  N=100  TunerSelectOption=Transfer Function Based (PID Tuner App)  InitialConditionSource=internal  InitialConditionForIntegrator=0  InitialConditionForFilter=0  DifferentiatorICPrevScaledInput=0  ExternalReset=none  TrackingMode=off  Kt=1  LimitOutput=off  SatLimitsSource=internal  UpperSaturationLimit=inf  LowerSaturationLimit=-inf  LinearizeAsGain=on  AntiWindupMode=none  Kb=1  POutMin=[]  POutMax=[]  IOutMin=[]  IOutMax=[]  DOutMin=[]  DOutMax=[]  NOutMin=[]  NOutMax=[]  SumOutMin=[]  SumOutMax=[]  SaturationOutMin=[]  SaturationOutMax=[]  PParamMin=[]  PParamMax=[]  IParamMin=[]  IParamMax=[]  DParamMin=[]  DParamMax=[]  NParamMin=[]  NParamMax=[]  KbParamMin=[]  KbParamMax=[]  KtParamMin=[]  KtParamMax=[]  KbOutMin=[]  KbOutMax=[]  KtOutMin=[]  KtOutMax=[]  IntegratorOutMin=[]  IntegratorOutMax=[]  FilterOutMin=[]  FilterOutMax=[]  SumI1OutMin=[]  SumI1OutMax=[]  SumI2OutMin=[]  SumI2OutMax=[]  SumI3OutMin=[]  SumI3OutMax=[]  SumI4OutMin=[]  SumI4OutMax=[]  SumDOutMin=[]  SumDOutMax=[]  DifferentiatorOutMin=[]  DifferentiatorOutMax=[]  FilterDiffOutCoefMin=[]  FilterDiffOutCoefMax=[]  ReciprocalOutMin=[]  ReciprocalOutMax=[]  SumDenOutMin=[]  SumDenOutMax=[]  SumNumOutMin=[]  SumNumOutMax=[]  DivideOutMin=[]  DivideOutMax=[]  UdiffTsProdOutMin=[]  UdiffTsProdOutMax=[]  NTsProdOutMin=[]  NTsProdOutMax=[]  UintegralTsProdOutMin=[]  UintegralTsProdOutMax=[]  UngainTsProdOutMin=[]  UngainTsProdOutMax=[]  IntegratorContinuousStateAttributes=''  IntegratorStateMustResolveToSignalObject=off  IntegratorRTWStateStorageClass=Auto  FilterContinuousStateAttributes=''  FilterStateMustResolveToSignalObject=off  FilterRTWStateStorageClass=Auto  ParallelPVariant=InternalParameters  IdealPVariant=Disabled  IVariant=InternalParameters  DVariant=Disabled  IntegratorVariant=Continuous  SatVariant=Disabled  AWVariant=Passthrough  PCopyVariant=Disabled  TRVariant=Disabled  FdbkBlocksVariant=Forward  IdealPFdbkVariant=Disabled  SatFdbkVariant=Disabled  DerivativeFilterVariant=Disabled  NVariant=Disabled  NCopyVariant=Disabled_SignalSpec  FilterICVariant=Disabled  IntegratorICVariant=InternalICs  ExternalResetVariant=Disabled  TRSumVariant=Passthrough  SumFdbkVariant=Disabled  SumVariant=Sum_PI  TsampFilterVariant=InternalTs  TsampNgainVariant=Passthrough  TsampIntegralVariant=Passthrough  ExternalSaturationOutDataTypeStr=Inherit: Same as second input
  PID Controller1 : pid_lib/PID Controller  Controller=PI  Form=Parallel  TimeDomain=Continuous-time  UseExternalTs=off  SampleTime=-1  IntegratorMethod=Forward Euler  FilterMethod=Forward Euler  ControllerParametersSource=internal  P=0.043  I=0.65  D=0  UseFilter=on  N=100  TunerSelectOption=Transfer Function Based (PID Tuner App)  InitialConditionSource=internal  InitialConditionForIntegrator=0  InitialConditionForFilter=0  DifferentiatorICPrevScaledInput=0  ExternalReset=none  TrackingMode=off  Kt=1  LimitOutput=off  SatLimitsSource=internal  UpperSaturationLimit=inf  LowerSaturationLimit=-inf  LinearizeAsGain=on  AntiWindupMode=none  Kb=1  POutMin=[]  POutMax=[]  IOutMin=[]  IOutMax=[]  DOutMin=[]  DOutMax=[]  NOutMin=[]  NOutMax=[]  SumOutMin=[]  SumOutMax=[]  SaturationOutMin=[]  SaturationOutMax=[]  PParamMin=[]  PParamMax=[]  IParamMin=[]  IParamMax=[]  DParamMin=[]  DParamMax=[]  NParamMin=[]  NParamMax=[]  KbParamMin=[]  KbParamMax=[]  KtParamMin=[]  KtParamMax=[]  KbOutMin=[]  KbOutMax=[]  KtOutMin=[]  KtOutMax=[]  IntegratorOutMin=[]  IntegratorOutMax=[]  FilterOutMin=[]  FilterOutMax=[]  SumI1OutMin=[]  SumI1OutMax=[]  SumI2OutMin=[]  SumI2OutMax=[]  SumI3OutMin=[]  SumI3OutMax=[]  SumI4OutMin=[]  SumI4OutMax=[]  SumDOutMin=[]  SumDOutMax=[]  DifferentiatorOutMin=[]  DifferentiatorOutMax=[]  FilterDiffOutCoefMin=[]  FilterDiffOutCoefMax=[]  ReciprocalOutMin=[]  ReciprocalOutMax=[]  SumDenOutMin=[]  SumDenOutMax=[]  SumNumOutMin=[]  SumNumOutMax=[]  DivideOutMin=[]  DivideOutMax=[]  UdiffTsProdOutMin=[]  UdiffTsProdOutMax=[]  NTsProdOutMin=[]  NTsProdOutMax=[]  UintegralTsProdOutMin=[]  UintegralTsProdOutMax=[]  UngainTsProdOutMin=[]  UngainTsProdOutMax=[]  IntegratorContinuousStateAttributes=''  IntegratorStateMustResolveToSignalObject=off  IntegratorRTWStateStorageClass=Auto  FilterContinuousStateAttributes=''  FilterStateMustResolveToSignalObject=off  FilterRTWStateStorageClass=Auto  ParallelPVariant=InternalParameters  IdealPVariant=Disabled  IVariant=InternalParameters  DVariant=Disabled  IntegratorVariant=Continuous  SatVariant=Disabled  AWVariant=Passthrough  PCopyVariant=Disabled  TRVariant=Disabled  FdbkBlocksVariant=Forward  IdealPFdbkVariant=Disabled  SatFdbkVariant=Disabled  DerivativeFilterVariant=Disabled  NVariant=Disabled  NCopyVariant=Disabled_SignalSpec  FilterICVariant=Disabled  IntegratorICVariant=InternalICs  ExternalResetVariant=Disabled  TRSumVariant=Passthrough  SumFdbkVariant=Disabled  SumVariant=Sum_PI  TsampFilterVariant=InternalTs  TsampNgainVariant=Passthrough  TsampIntegralVariant=Passthrough  ExternalSaturationOutDataTypeStr=Inherit: Same as second input
  PID Controller2 : pid_lib/PID Controller  Controller=PI  Form=Parallel  TimeDomain=Continuous-time  UseExternalTs=off  SampleTime=-1  IntegratorMethod=Forward Euler  FilterMethod=Forward Euler  ControllerParametersSource=internal  P=0.45  I=14800  D=0  UseFilter=on  N=100  TunerSelectOption=Transfer Function Based (PID Tuner App)  InitialConditionSource=internal  InitialConditionForIntegrator=0  InitialConditionForFilter=0  DifferentiatorICPrevScaledInput=0  ExternalReset=none  TrackingMode=off  Kt=1  LimitOutput=off  SatLimitsSource=internal  UpperSaturationLimit=inf  LowerSaturationLimit=-inf  LinearizeAsGain=on  AntiWindupMode=none  Kb=1  POutMin=[]  POutMax=[]  IOutMin=[]  IOutMax=[]  DOutMin=[]  DOutMax=[]  NOutMin=[]  NOutMax=[]  SumOutMin=[]  SumOutMax=[]  SaturationOutMin=[]  SaturationOutMax=[]  PParamMin=[]  PParamMax=[]  IParamMin=[]  IParamMax=[]  DParamMin=[]  DParamMax=[]  NParamMin=[]  NParamMax=[]  KbParamMin=[]  KbParamMax=[]  KtParamMin=[]  KtParamMax=[]  KbOutMin=[]  KbOutMax=[]  KtOutMin=[]  KtOutMax=[]  IntegratorOutMin=[]  IntegratorOutMax=[]  FilterOutMin=[]  FilterOutMax=[]  SumI1OutMin=[]  SumI1OutMax=[]  SumI2OutMin=[]  SumI2OutMax=[]  SumI3OutMin=[]  SumI3OutMax=[]  SumI4OutMin=[]  SumI4OutMax=[]  SumDOutMin=[]  SumDOutMax=[]  DifferentiatorOutMin=[]  DifferentiatorOutMax=[]  FilterDiffOutCoefMin=[]  FilterDiffOutCoefMax=[]  ReciprocalOutMin=[]  ReciprocalOutMax=[]  SumDenOutMin=[]  SumDenOutMax=[]  SumNumOutMin=[]  SumNumOutMax=[]  DivideOutMin=[]  DivideOutMax=[]  UdiffTsProdOutMin=[]  UdiffTsProdOutMax=[]  NTsProdOutMin=[]  NTsProdOutMax=[]  UintegralTsProdOutMin=[]  UintegralTsProdOutMax=[]  UngainTsProdOutMin=[]  UngainTsProdOutMax=[]  IntegratorContinuousStateAttributes=''  IntegratorStateMustResolveToSignalObject=off  IntegratorRTWStateStorageClass=Auto  FilterContinuousStateAttributes=''  FilterStateMustResolveToSignalObject=off  FilterRTWStateStorageClass=Auto  ParallelPVariant=InternalParameters  IdealPVariant=Disabled  IVariant=InternalParameters  DVariant=Disabled  IntegratorVariant=Continuous  SatVariant=Disabled  AWVariant=Passthrough  PCopyVariant=Disabled  TRVariant=Disabled  FdbkBlocksVariant=Forward  IdealPFdbkVariant=Disabled  SatFdbkVariant=Disabled  DerivativeFilterVariant=Disabled  NVariant=Disabled  NCopyVariant=Disabled_SignalSpec  FilterICVariant=Disabled  IntegratorICVariant=InternalICs  ExternalResetVariant=Disabled  TRSumVariant=Passthrough  SumFdbkVariant=Disabled  SumVariant=Sum_PI  TsampFilterVariant=InternalTs  TsampNgainVariant=Passthrough  TsampIntegralVariant=Passthrough  ExternalSaturationOutDataTypeStr=Inherit: Same as second input
  PWM Generator (DC-DC) : spsPWMGeneratorDCDCLib/PWM Generator (DC-DC)  Fsw=20000  Ts=0
  PWM Generator (DC-DC)1 : spsPWMGeneratorDCDCLib/PWM Generator (DC-DC)  Fsw=20000  Ts=0
  Saturation : Saturate  UpperLimit=1  LowerLimit=0
  Saturation1 : Saturate  UpperLimit=1  LowerLimit=0
  Sum{,1..3} (4 alike) : Sum  Inputs=|+-
  Sum4 : Sum  Inputs=|++
  Q1_Bat : Outport
  Q2_Bat : Outport  Port=2
  Q1_SC : Outport  Port=3
  Q2_SC : Outport  Port=4
  wires:
  Sum1/1 -> PID Controller1/1, Sum4/2
  PWM Generator (DC-DC)/1 -> Logical Operator1/1, Q2_Bat/1
  I_Bat/1 -> Sum1/2
  I_SC/1 -> Sum2/2
  Sum2/1 -> PID Controller2/1
  Logical Operator1/1 -> Q1_Bat/1
  Sum/1 -> PID Controller/1
  VDC_ref/1 -> Sum/1
  V_DC/1 -> Sum/2
  V_Bat/1 -> Divide/1
  "V_SC "/1 -> Divide/2
  Logical Operator4/1 -> Q1_SC/1
  PWM Generator (DC-DC)1/1 -> Q2_SC/1, Logical Operator4/1
  PID Controller/1 -> First-Order Filter/1, Sum3/1
  Sum3/1 -> Sum4/1
  Divide1/1 -> Sum2/1
  Divide/1 -> Divide1/2
  Sum4/1 -> Divide1/1
  PID Controller2/1 -> Saturation/1
  Saturation/1 -> PWM Generator (DC-DC)1/1
  PID Controller1/1 -> Saturation1/1
  Saturation1/1 -> PWM Generator (DC-DC)/1
  First-Order Filter/1 -> Sum1/1, Sum3/2

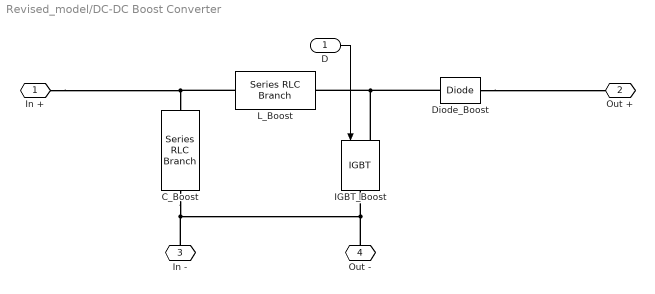
== system Revised_model/DC-DC Boost Converter ==
  D : Inport
  C_Boost : spsSeriesRLCBranchLib/Series RLC Branch  LConnTagsString=__new0  RConnTagsString=__new0  BranchType=C  Resistance=0.01  Inductance=1e-3  SetiL0=off  InitialCurrent=0  Capacitance=2200e-6  Setx0=off  InitialVoltage=0  Measurements=None
  Diode_Boost : spsDiodeLib/Diode  Ron=1e-4  Lon=0  Vf=0  IC=0  UseSnubber=off  Rs=inf  Cs=inf  Measurements=off
  IGBT_Boost : spsIGBTLib/IGBT  Ron=0.001  Lon=0  Vf=0  Tf=0  Tt=0  IC=0  Rs=1e5  Cs=inf  Measurements=off
  L_Boost : spsSeriesRLCBranchLib/Series RLC Branch  LConnTagsString=__new0  RConnTagsString=__new0  BranchType=RL  Resistance=0.05  Inductance=0.352e-3  SetiL0=off  InitialCurrent=0  Capacitance=1e-6  Setx0=off  InitialVoltage=0  Measurements=None
  In + : PMIOPort  Side=Left
  Out + : PMIOPort  Port=2  Side=Right
  In - : PMIOPort  Port=3  Side=Left
  Out - : PMIOPort  Port=4  Side=Right
  wires:
  D/1 -> IGBT_Boost/1
  connections:
  IGBT_Boost/LConn1 -- Diode_Boost/LConn1 -- L_Boost/RConn1
  Diode_Boost/RConn1 -- Out +/RConn1
  L_Boost/LConn1 -- In +/RConn1 -- C_Boost/LConn1
  C_Boost/RConn1 -- In -/RConn1 -- Out -/RConn1 -- IGBT_Boost/RConn1
